simulink model "shoukongkalman_total"  (R2024b)
settings: Solver=FixedStepAuto  StartTime=0.0  StopTime=10.0  FixedStep=1  RelTol=1e-3
settings Model: Creator=54238  LastModifiedBy=54238

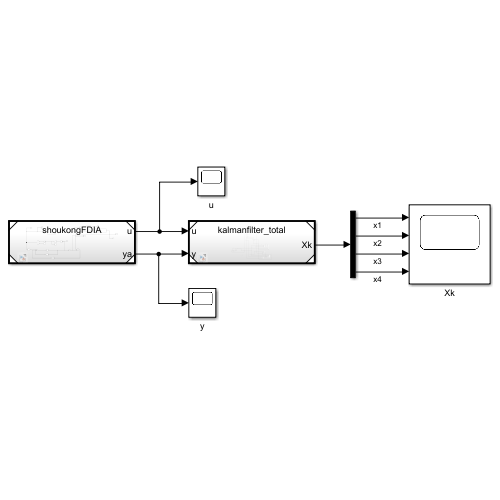
[thumbnail: Simulink's stored preview of the top-level diagram]
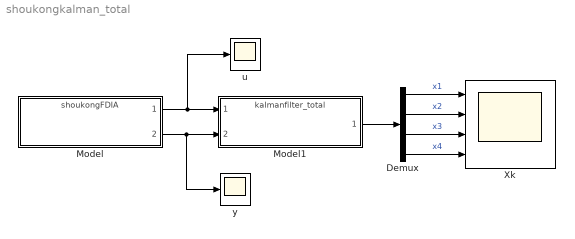
== system shoukongkalman_total ==
  Demux : Demux
  Model : ModelReference  ModelNameDialog=shoukongFDIA.slx  SimulationMode=Normal  ModelReferenceVersion=1.19
  Model1 : ModelReference  ModelNameDialog=kalmanfilter_total.slx  SimulationMode=Normal  ModelReferenceVersion=1.2
  Xk : Scope  NumInputPorts=4
  u : Scope
  y : Scope
  wires:
  Model/1 -> Model1/1, u/1
  Model/2 -> Model1/2, y/1
  Model1/1 -> Demux/1
  Demux/1 -> Xk/1  "x1"
  Demux/2 -> Xk/2  "x2"
  Demux/3 -> Xk/3  "x3"
  Demux/4 -> Xk/4  "x4"
